simulink model "DeadZoneBlockSimulink"  (R2024a)
settings: Solver=FixedStepDiscrete  StartTime=0.0  StopTime=10.0  FixedStep=0.1  RelTol=1e-3
libraries: simulink x1
settings Model: Creator=prabo  LastModifiedBy=prabo

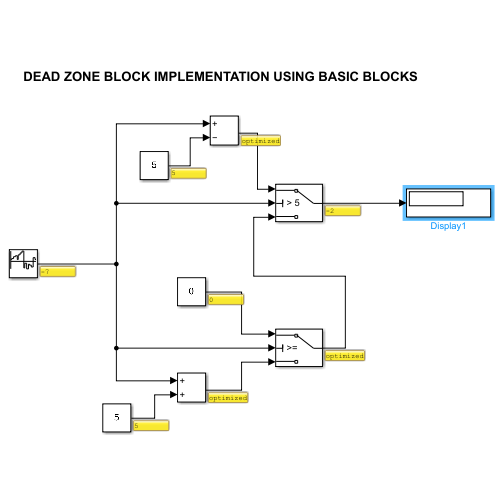
[thumbnail: Simulink's stored preview of the top-level diagram]
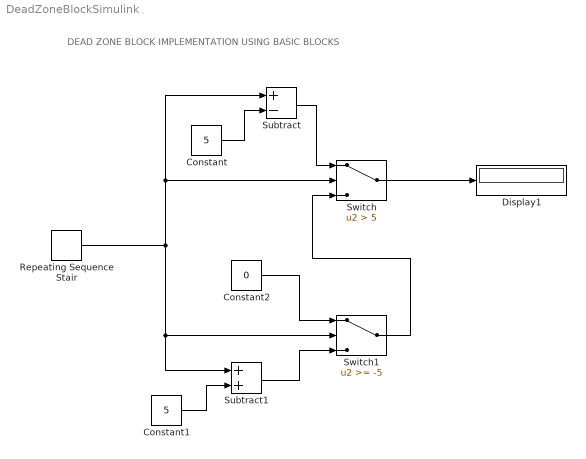
== system DeadZoneBlockSimulink ==
  note: DEAD ZONE BLOCK IMPLEMENTATION USING BASIC BLOCKS
  Constant : Constant  Value=5
  Constant1 : Constant  Value=5
  Constant2 : Constant  Value=0
  Display1 : Display
  Repeating Sequence Stair : simulink/Sources/Repeating Sequence Stair  OutValues=[3 5 7 8 3 9 12 15 -9 -2 -10 -3 -5 -7 6 3].'  tsamp=-1  OutMin=[]  OutMax=[]  OutDataTypeStr=double  OutputDataTypeScalingMode=double  OutDataType=fixdt(0,8)  ConRadixGroup=Best Precision: Vector-wise  OutScaling=2^-12
  Subtract : Sum  Inputs=+-
  Subtract1 : Sum
  Switch : Switch  Criteria=u2 > Threshold  Threshold=5  SaturateOnIntegerOverflow=off  InputSameDT=off
  Switch1 : Switch  Threshold=-5  SaturateOnIntegerOverflow=off  InputSameDT=off
  wires:
  Repeating Sequence Stair/1 -> Subtract/1, Switch/2, Subtract1/1, Switch1/2
  Constant/1 -> Subtract/2
  Subtract/1 -> Switch/1
  Switch1/1 -> Switch/3
  Switch/1 -> Display1/1
  Constant2/1 -> Switch1/1
  Constant1/1 -> Subtract1/2
  Subtract1/1 -> Switch1/3
